simulink model "ADRC_Implementation_2017"  (R2017a)
settings: Solver=ode4  StartTime=0.0  StopTime=2  FixedStep=0.01  RelTol=1e-3
settings Model: Creator=rastronaut  LastModifiedBy=rastronaut

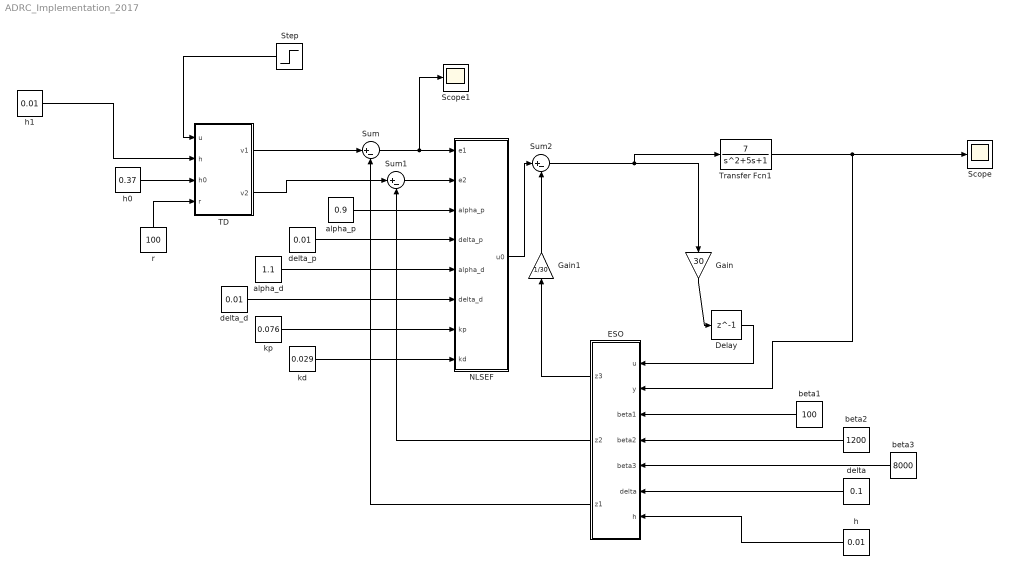
== system ADRC_Implementation_2017 ==
  Delay : Delay  DelayLength=1  InitialCondition=0
  ESO : MATLAB Function  TreatAsAtomicUnit=on
  Gain : Gain  Gain=30
  Gain1 : Gain  Gain=1/30
  NLSEF : MATLAB Function  TreatAsAtomicUnit=on
  Scope : Scope
  Scope1 : Scope
  Step : Step  SampleTime=0
  Sum : Sum  Inputs=|+-
  Sum1 : Sum  Inputs=|+-
  Sum2 : Sum  Inputs=|+-
  "TD " : MATLAB Function  TreatAsAtomicUnit=on
  Transfer Fcn1 : TransferFcn  Numerator=[7]  Denominator="[1  5  1]"
  alpha_d : Constant  Value=1.1
  alpha_p : Constant  Value=0.9
  beta1 : Constant  Value=100
  beta2 : Constant  Value=1200
  beta3 : Constant  Value=8000
  delta : Constant  Value=0.1
  delta_d : Constant  Value=0.01
  delta_p : Constant  Value=0.01
  h : Constant  Value=0.01
  h0 : Constant  Value=0.37
  h1 : Constant  Value=0.01
  kd : Constant  Value=0.029
  kp : Constant  Value=0.076
  r : Constant  Value=100
  wires:
  Gain1/1 -> Sum2/2
  "TD "/1(v1) -> Sum/1
  "TD "/2(v2) -> Sum1/1
  ESO/3(z1) -> Sum/2
  ESO/2(z2) -> Sum1/2
  ESO/1(z3) -> Gain1/1
  NLSEF/1(u0) -> Sum2/1
  Sum/1 -> Scope1/1, NLSEF/1(e1)
  Sum1/1 -> NLSEF/2(e2)
  Transfer Fcn1/1 -> Scope/1, ESO/2(y)
  Step/1 -> "TD "/1(u)
  beta1/1 -> ESO/3(beta1)
  beta2/1 -> ESO/4(beta2)
  beta3/1 -> ESO/5(beta3)
  delta/1 -> ESO/6(delta)
  alpha_p/1 -> NLSEF/3(alpha_p)
  delta_p/1 -> NLSEF/4(delta_p)
  alpha_d/1 -> NLSEF/5(alpha_d)
  delta_d/1 -> NLSEF/6(delta_d)
  h0/1 -> "TD "/3(h0)
  r/1 -> "TD "/4(r)
  kp/1 -> NLSEF/7(kp)
  kd/1 -> NLSEF/8(kd)
  Sum2/1 -> Gain/1, Transfer Fcn1/1
  Delay/1 -> ESO/1(u)
  Gain/1 -> Delay/1
  h/1 -> ESO/7(h)
  h1/1 -> "TD "/2(h)

== matlab function ADRC_Implementation_2017/ESO ==
  settings: updateMethod=DISCRETE
  data: u input; z3 output; z2 output; y input; z1 output; beta1 input; beta2 input; beta3 input; delta input; h input
function [z3,z2,z1] = ESO(u,y,beta1,beta2,beta3,delta,h)
persistent z1_old;
persistent z2_old;
persistent z3_old;
persistent u_old;
persistent y_old;

if isempty(z1_old)
     z1_old=0;
end
if isempty(z2_old)
     z2_old=0;
end
if isempty(z3_old)
     z3_old=0;
end
if isempty(u_old)
     u_old=0;
end
if isempty(y_old)
     y_old=0;
end


e = z1_old - y_old;
z1 = z1_old + h*(z2_old - beta1*e);
z2 = z2_old + h*(z3_old - beta2*fal(e, 0.5, delta) + u_old);
z3 = z3_old - h*beta3*fal(e, 0.25, delta);

z1_old = z1;
z2_old = z2;
z3_old = z3;
u_old = u;
y_old = y;

end

== matlab function ADRC_Implementation_2017/TD  ==
  settings: updateMethod=DISCRETE
  data: u input; v1 output; v2 output; h input; h0 input; r input
function [v1,v2] = TD(u,h,h0,r)
persistent v1_old;
persistent v2_old;
persistent u_old;
if isempty(v1_old)
     v1_old=0;
end
if isempty(v2_old)
     v2_old=0;
end
if isempty(u_old)
     u_old=0;
end
v1=v1_old+h*v2_old;
v2=v2_old+h*fhan(v1_old-u_old,v2_old,r,h0);
v1_old = v1;
v2_old = v2;
u_old = u;  
end

== matlab function ADRC_Implementation_2017/NLSEF ==
  data: e1 input; u0 output; e2 input; alpha_p input; delta_p input; alpha_d input; delta_d input; kp input; kd input
function u0 = NLSEF(e1,e2,alpha_p,delta_p,alpha_d,delta_d,kp,kd)

u0 = kp*fal(e1, alpha_p, delta_p) + kd*fal(e2, alpha_d, delta_d);

end
